simulink subsystem "ForwardingAndHazardDetectionUnit"  (R2024b)
settings: Solver=VariableStepAuto  StartTime=0.0  StopTime=10.0  RelTol=1e-3
settings Model: Creator=stefano  LastModifiedBy=stefano

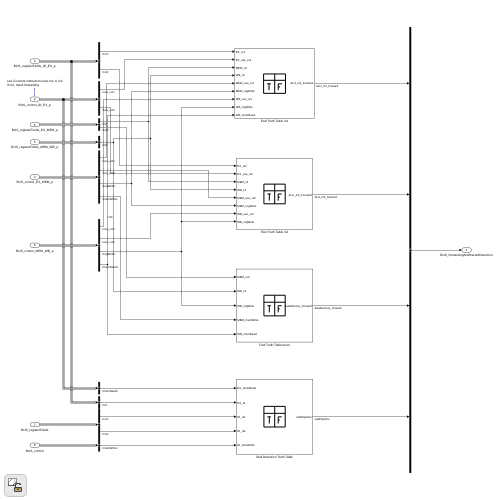
[thumbnail: Simulink's stored preview of the top-level diagram]
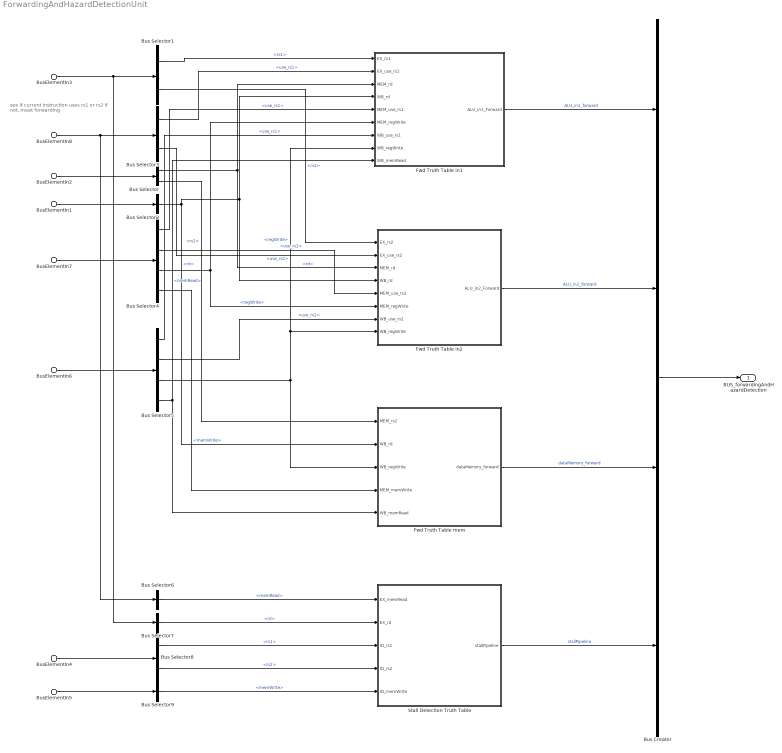
== system ForwardingAndHazardDetectionUnit ==
  note: see if current instruction uses rs1 or rs2
      | if not, mask forwarding
  BusElementIn1 : Inport  PortName=BUS_toFwdUnit_MEM_WB_p  Element=BUS_registerFields_MEM_WB_p
  BusElementIn2 : Inport  PortName=BUS_toFwdUnit_MEM_WB_p  Element=BUS_registerFields_EX_MEM_p
  BusElementIn3 : Inport  PortName=BUS_toFwdUnit_MEM_WB_p  Element=BUS_registerFields_ID_EX_p
  BusElementIn4 : Inport  PortName=BUS_toFwdUnit_MEM_WB_p  Element=BUS_registerFields
  BusElementIn5 : Inport  PortName=BUS_toFwdUnit_MEM_WB_p  Element=BUS_control
  BusElementIn6 : Inport  PortName=BUS_toFwdUnit_MEM_WB_p  Element=BUS_control_MEM_WB_p
  BusElementIn7 : Inport  PortName=BUS_toFwdUnit_MEM_WB_p  Element=BUS_control_EX_MEM_p
  BusElementIn8 : Inport  PortName=BUS_toFwdUnit_MEM_WB_p  Element=BUS_control_ID_EX_p
  Bus Creator : BusCreator  Inputs=4
  Bus Selector : BusSelector  OutputSignals=rd,rs2
  Bus Selector1 : BusSelector  OutputSignals=rs1,rs2
  Bus Selector2 : BusSelector  OutputSignals=rd
  Bus Selector3 : BusSelector  OutputSignals=use_rs1,use_rs2
  Bus Selector4 : BusSelector  OutputSignals=use_rs1,use_rs2,regWrite,memWrite
  Bus Selector5 : BusSelector  OutputSignals=use_rs1,use_rs2,regWrite,memRead
  Bus Selector6 : BusSelector  OutputSignals=memRead
  Bus Selector7 : BusSelector  OutputSignals=rd
  Bus Selector8 : BusSelector  OutputSignals=rs1,rs2
  Bus Selector9 : BusSelector  OutputSignals=memWrite
  Fwd Truth Table in1 : Truth Table  TreatAsAtomicUnit=on
  Fwd Truth Table in2 : Truth Table  TreatAsAtomicUnit=on
      settings: PortSchema="{\"entries\":[{\"content\":{\"sides\":[{\"content\":{\"connectorIds\":[\"In2\",\"In3\",\"In4\",\"In5\",\"In6\",\"In7\",\"In1\",\"In8\"]},\"type\":\"ConnectorPlacement.EquallySpacedRectSide\",\"uuid\":\"3767e3cd-f9a3-4376-8cef-5f6f85c19d3e\"},{\"content\":{\"connectorIds\":[\"Out1\"],\"side\":\"RIGHT\"},\"type\":\"ConnectorPlacement.EquallySpacedRectSide\",\"uuid\":\"c978069b-1b3e-43b4-8124-5d67bb74c2ad\"},{\"content\":{\"side\":\"TOP\"},\"type\":\"ConnectorPlacement.EquallySpacedRectSide\",\"uuid\":\"3ad345e6-fd8a-4a16-90ae-dd2366ba6706\"},{\"content\":{\"side\":\"BOTTOM\"},\"type\":\"ConnectorPlacement.EquallySpacedRectSide\",\"uuid\":\"22acd140-9183-4979-a82a-291b6442d565\"}]},\"type\":\"ConnectorPlacement.EquallySpacedConnector\",\"uuid\":\"0d6623b5-08cd-48c6-aa29-bb6800c54a2e\"}],\"packageUris\":[\"http://schema.mathworks.com/mf0/Connector/R2020b\"],\"version\":\"1.0\"}"
  Fwd Truth Table mem : Truth Table  TreatAsAtomicUnit=on
  Stall Detection Truth Table : Truth Table  TreatAsAtomicUnit=on
  BUS_forwardingAndHazardDetection : Outport
  wires:
  BusElementIn2/1 -> Bus Selector/1
  BusElementIn3/1 -> Bus Selector1/1, Bus Selector7/1
  BusElementIn1/1 -> Bus Selector2/1
  BusElementIn8/1 -> Bus Selector3/1, Bus Selector6/1
  BusElementIn7/1 -> Bus Selector4/1
  Bus Selector2/1 -> Fwd Truth Table mem/2(WB_rd), Fwd Truth Table in1/4(WB_rd), Fwd Truth Table in2/5(WB_rd)  "<rd>"
  Bus Selector/1 -> Fwd Truth Table in1/3(MEM_rd), Fwd Truth Table in2/4(MEM_rd)  "<rd>"
  Bus Selector1/1 -> Fwd Truth Table in1/1(EX_rs1)  "<rs1>"
  Bus Selector3/1 -> Fwd Truth Table in1/2(EX_use_rs1)  "<use_rs1>"
  Fwd Truth Table in2/1(ALU_in2_Forward) -> Bus Creator/2  "ALU_in2_forward"
  Bus Selector4/1 -> Fwd Truth Table in1/5(MEM_use_rs1)  "<use_rs1>"
  Bus Selector4/3 -> Fwd Truth Table in1/6(MEM_regWrite), Fwd Truth Table in2/7(MEM_regWrite)  "<regWrite>"
  BusElementIn6/1 -> Bus Selector5/1
  Bus Selector5/1 -> Fwd Truth Table in1/7(WB_use_rs1)  "<use_rs1>"
  Bus Selector5/3 -> Fwd Truth Table mem/3(WB_regWrite), Fwd Truth Table in2/8(WB_regWrite), Fwd Truth Table in1/8(WB_regWrite)  "<regWrite>"
  Fwd Truth Table in1/1(ALU_in1_Forward) -> Bus Creator/1  "ALU_in1_forward"
  Bus Selector1/2 -> Fwd Truth Table in2/2(EX_rs2)  "<rs2>"
  Bus Selector3/2 -> Fwd Truth Table in2/3(EX_use_rs2)  "<use_rs2>"
  Bus Selector4/2 -> Fwd Truth Table in2/6(MEM_use_rs2)  "<use_rs2>"
  Bus Selector5/2 -> Fwd Truth Table in2/1(WB_use_rs2)  "<use_rs2>"
  Fwd Truth Table mem/1(dataMemory_forward) -> Bus Creator/3  "dataMemory_forward"
  Bus Selector4/4 -> Fwd Truth Table mem/4(MEM_memWrite)  "<memWrite>"
  Bus Selector/2 -> Fwd Truth Table mem/1(MEM_rs2)  "<rs2>"
  Bus Selector5/4 -> Fwd Truth Table mem/5(WB_memRead), Fwd Truth Table in1/9(WB_memRead)  "<memRead>"
  Bus Selector6/1 -> Stall Detection Truth Table/1(EX_memRead)  "<memRead>"
  BusElementIn4/1 -> Bus Selector8/1
  Bus Selector8/1 -> Stall Detection Truth Table/3(ID_rs1)  "<rs1>"
  Bus Selector8/2 -> Stall Detection Truth Table/4(ID_rs2)  "<rs2>"
  Bus Selector7/1 -> Stall Detection Truth Table/2(EX_rd)  "<rd>"
  Stall Detection Truth Table/1(stallPipeline) -> Bus Creator/4  "stallPipeline"
  BusElementIn5/1 -> Bus Selector9/1
  Bus Selector9/1 -> Stall Detection Truth Table/5(ID_memWrite)  "<memWrite>"
  Bus Creator/1 -> BUS_forwardingAndHazardDetection/1

== matlab function ForwardingAndHazardDetectionUnit/Fwd Truth Table in1 ==
  data: EX_rs1 input fixdt(0,5,0); EX_use_rs1 input boolean; MEM_rd input fixdt(0,5,0); WB_rd input fixdt(0,5,0); MEM_use_rs1 input; MEM_regWrite input boolean; WB_use_rs1 input; WB_regWrite input boolean; ALU_in1_Forward output fixdt(0,2,0); WB_memRead input
function ALU_in1_Forward = fcn(EX_rs1, EX_use_rs1, MEM_rd, WB_rd, MEM_use_rs1, MEM_regWrite, WB_use_rs1, WB_regWrite, WB_memRead)

aVarTruthTableCondition_1 = false;
aVarTruthTableCondition_2 = false;
aVarTruthTableCondition_3 = false;


% EX hazard rs1 ALU

aVarTruthTableCondition_1 = logical(MEM_regWrite == true &&  MEM_rd  ~= 0 &&  MEM_rd == EX_rs1 &&  EX_use_rs1 == true);

% MEM hazard rs1 ALU

aVarTruthTableCondition_2 = logical(WB_regWrite == true &&  WB_rd  ~= 0 &&  WB_rd == EX_rs1 &&  WB_memRead == false && EX_use_rs1 == true);

% MEM hazard rs1 memory

aVarTruthTableCondition_3 = logical(WB_regWrite == true &&  WB_rd  ~= 0 &&  WB_rd == EX_rs1 &&  WB_memRead == true && EX_use_rs1 == true);

if (aVarTruthTableCondition_1)
    in1_MEM();
elseif (aVarTruthTableCondition_2)
    in1_WB();
elseif (aVarTruthTableCondition_3)
    in1_WB_mem();
else % Default
    no_fwd();
end

function no_fwd()



ALU_in1_Forward = 0;

function in1_MEM()

% ALU_in1 from MEM ALU

ALU_in1_Forward = 2;

function in1_WB()

% ALU_in1 from WB ALU

ALU_in1_Forward = 1;

function in1_WB_mem()

% ALU_in1 from WB memory

ALU_in1_Forward = 3;

== matlab function ForwardingAndHazardDetectionUnit/Fwd Truth Table in2 ==
  data: WB_use_rs2 input; EX_rs2 input fixdt(0,5,0); EX_use_rs2 input boolean; MEM_rd input fixdt(0,5,0); WB_rd input fixdt(0,5,0); ALU_in2_Forward output fixdt(0,2,0); MEM_use_rs2 input; MEM_regWrite input boolean; WB_regWrite input boolean
function ALU_in2_Forward = fcn(WB_use_rs2, EX_rs2, EX_use_rs2, MEM_rd, WB_rd, MEM_use_rs2, MEM_regWrite, WB_regWrite)

aVarTruthTableCondition_1 = false;
aVarTruthTableCondition_2 = false;


% EX hazard rs2

aVarTruthTableCondition_1 = logical(MEM_regWrite == true &&  MEM_rd  ~= 0 &&  MEM_rd == EX_rs2 &&  EX_use_rs2 == true);

% MEM hazard rs2

aVarTruthTableCondition_2 = logical(WB_regWrite == true &&  WB_rd  ~= 0 &&  WB_rd == EX_rs2 &&  EX_use_rs2 == true);

if (aVarTruthTableCondition_1)
    in2_MEM();
elseif (aVarTruthTableCondition_2)
    in2_WB();
else % Default
    no_fwd();
end

function no_fwd()



ALU_in2_Forward = 0;

function in2_MEM()

% ALU_in2 from MEM

ALU_in2_Forward = 2;

function in2_WB()

% ALU_in2 from WB

ALU_in2_Forward = 1;

== matlab function ForwardingAndHazardDetectionUnit/Fwd Truth Table mem ==
  data: MEM_rs2 input fixdt(0,5,0); WB_rd input fixdt(0,5,0); dataMemory_forward output fixdt(0,2,0); WB_regWrite input boolean; MEM_memWrite input boolean; WB_memRead input
function dataMemory_forward = fcn(MEM_rs2, WB_rd, WB_regWrite, MEM_memWrite, WB_memRead)

aVarTruthTableCondition_1 = false;
aVarTruthTableCondition_2 = false;


% MEM hazard dataIn from ALU

aVarTruthTableCondition_1 = logical(WB_regWrite == true &&  WB_memRead == false &&  WB_rd  ~= 0 &&  WB_rd == MEM_rs2 &&  MEM_memWrite == true);

% MEM hazard dataIn from read

aVarTruthTableCondition_2 = logical(WB_regWrite == true &&  WB_memRead == true &&  WB_rd  ~= 0 &&  WB_rd == MEM_rs2 &&  MEM_memWrite == true);

if (aVarTruthTableCondition_1)
    dataMemory_dataIn_WB_ALU();
elseif (aVarTruthTableCondition_2)
    dataMemory_dataIn_WB_MEM();
else % Default
    no_fwd();
end

function no_fwd()



dataMemory_forward = 0;

function dataMemory_dataIn_WB_ALU()

% dataMemory_dataIn from WB

dataMemory_forward = 1;

function dataMemory_dataIn_WB_MEM()

% dataMemory_dataIn from mem read

dataMemory_forward = 2;

== matlab function ForwardingAndHazardDetectionUnit/Stall Detection Truth Table ==
  data: EX_memRead input boolean; EX_rd input fixdt(0,5,0); ID_rs1 input fixdt(0,5,0); ID_rs2 input fixdt(0,5,0); stallPipeline output boolean; ID_memWrite input boolean
function stallPipeline = fcn(EX_memRead, EX_rd, ID_rs1, ID_rs2, ID_memWrite)

aVarTruthTableCondition_1 = false;


% Register read after same register write

aVarTruthTableCondition_1 = logical(EX_memRead == true &&  EX_rd ~= 0 &&  ID_memWrite == false && (EX_rd == ID_rs1 || EX_rd == ID_rs2));

if (aVarTruthTableCondition_1)
    stall();
else % Default
    no_stall();
end

function no_stall()



stallPipeline = false;

function stall()

% stall pipeline

stallPipeline = true;
